simulink model "task3"  (R2023a)
settings: Solver=VariableStepAuto  StartTime=0.0  StopTime=20.0  RelTol=1e-8
settings Model: Creator=vasil  LastModifiedBy=vasil

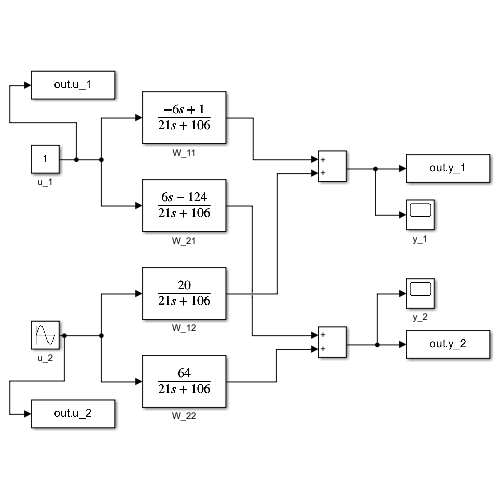
[thumbnail: Simulink's stored preview of the top-level diagram]
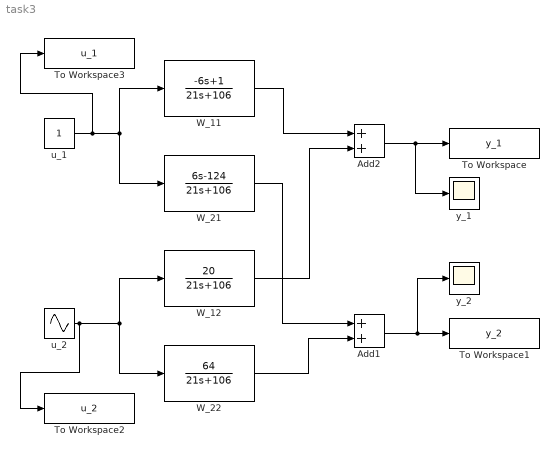
== system task3 ==
  Add1 : Sum
  Add2 : Sum
  To Workspace : ToWorkspace  VariableName=y_1  SaveFormat=Timeseries  SampleTime=-1
  To Workspace1 : ToWorkspace  VariableName=y_2  SaveFormat=Timeseries  SampleTime=-1
  To Workspace2 : ToWorkspace  VariableName=u_2  SaveFormat=Timeseries  SampleTime=-1
  To Workspace3 : ToWorkspace  VariableName=u_1  SaveFormat=Timeseries  SampleTime=-1
  W_11 : TransferFcn  Numerator=[-6 1]  Denominator=[21 106]
  W_12 : TransferFcn  Numerator=[20]  Denominator=[21 106]
  W_21 : TransferFcn  Numerator=[6 -124]  Denominator=[21 106]
  W_22 : TransferFcn  Numerator=[64]  Denominator=[21 106]
  u_1 : Constant
  u_2 : Sin  Amplitude=2  SampleTime=0
  y_1 : Scope
  y_2 : Scope
  wires:
  W_11/1 -> Add2/1
  W_12/1 -> Add2/2
  W_21/1 -> Add1/1
  W_22/1 -> Add1/2
  Add1/1 -> y_2/1, To Workspace1/1
  Add2/1 -> y_1/1, To Workspace/1
  u_1/1 -> To Workspace3/1, W_21/1, W_11/1
  u_2/1 -> To Workspace2/1, W_22/1, W_12/1
